simulink model "bbcontroller"  (R2014a)
settings: Solver=FixedStepDiscrete  StartTime=0.0  StopTime=10  FixedStep=0.01  RelTol=1e-3
settings Model: Creator=alexandru  LastModifiedBy=alexandru
settings DataIOCC: LimitDataPoints=off  SaveState=on  DSMLogging=off  InspectSignalLogs=on
settings HardwareCC: TargetBitPerLong=64  TargetBitPerPointer=64  TargetLongLongMode=on  TargetIntDivRoundTo=Zero  TargetEndianess=LittleEndian  TargetWordSize=64  TargetHWDeviceType=MATLAB Host  ProdEqTarget=off
settings RTWCC: SystemTargetFile=rsim.tlc  GenCodeOnly=on  PackageGeneratedCodeAndArtifacts=on  PackageName=idhp_model_heart_realtime  TemplateMakefile=rsim_default_tmf  Description=Rapid Simulation Target  ProcessScript=rsim_make_rtw_hook
settings RSimTargetCC: ERTMultiwordTypeDef=System defined  ERTMultiwordLength=256  EnableShiftOperators=on

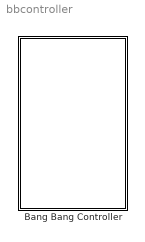
== system bbcontroller ==
  Bang Bang Controller : Stateflow chart  Priority=1  TreatAsAtomicUnit=on

== stateflow chart bbcontroller/Bang Bang Controller ==
  state BangBang
    state Heater [parallel]
      settings: executionOrder=3
      state Off
      state On
      (default) -> BangBang.Heater.Off
      BangBang.Heater.Off -> BangBang.Heater.Off [order 2] : after(T_INC,msec)[temp>-10.0]
          | {temp=temp-T_INC*0.004;}
      BangBang.Heater.Off -> BangBang.Heater.On [order 1] : HON
      BangBang.Heater.On -> BangBang.Heater.Off [order 1] : HOFF
      BangBang.Heater.On -> BangBang.Heater.On [order 2] : after(T_INC,msec)
          | {temp=temp+T_INC*0.04;}
    state Controller [parallel]
      settings: executionOrder=1
      state Off
      state On
      state Onp
      (default) -> BangBang.Controller.Off
      Onp -> BangBang.Controller.Off [order 1] : [temp>=25.0]
          | {send(FON,Led);
          | send(HOFF,Heater);}
      BangBang.Controller.On -> BangBang.Controller.Off [order 1] : after(T_OFF,msec)
          | {send(FON,Led);
          | send(HOFF,Heater);}
      BangBang.Controller.Off -> BangBang.Controller.On : after(T_ON, msec)[temp<25.0]
          | {send(FOFF,Led);
          | send(HON,Heater);}
      Onp -> BangBang.Controller.On [order 2] : [temp<25.0]
      BangBang.Controller.On -> Onp [order 2] : after(T_POLL,msec)
    state Led [parallel]
      settings: executionOrder=2
      state Flash_Off
      state Flash_On
      state Off
      Flash_Off -> Flash_On [order 2] : after(5,msec)
          | {dW(11,1);}
      (default) -> Flash_Off
      Flash_On -> Flash_Off [order 2] : after(5,msec)
          | {dW(11,0);}
      Flash_Off -> BangBang.Led.Off [order 1] : FOFF
          | {dW(11,0);}
      BangBang.Led.Off -> Flash_Off : FON
      Flash_On -> BangBang.Led.Off [order 1] : FOFF
          | {dW(11,0);}
  (default) -> BangBang
  data: stat function_output double; port function_input double; value function_input double; T_OFF local uint32 =20; T_ON local uint32 =40; temp local uint8 =20; T_POLL local uint32 =10; ref local double; T_INC local uint32 =100
  events: FOFF local EITHER_EDGE_EVENT; FON local EITHER_EDGE_EVENT; HOFF local FUNCTION_CALL_EVENT; HON local FUNCTION_CALL_EVENT
  function stat  = dW(port, value):
    | function stat  = dW(port, value)
    |     stat  = 0;
    | end
